simulink model "task4-Simulink"  (R2015b)
settings: Solver=VariableStepAuto  StartTime=0.0  StopTime=10.0  RelTol=1e-3
values from neighbouring files (symbols this model uses):
  J = 60*10^-7    (= 6e-06)    [All Tasks Compiled.m]
  Kemf = 4.555*10^(-3)*60/(2*pi)    (= 0.043497045947)    [All Tasks Compiled.m]
  Km = 43.5*10^-3    (= 0.0435)    [All Tasks Compiled.m]
  R = 1.45    [All Tasks Compiled.m]
settings Model: Creator=daniella.a  LastModifiedBy=daniella.a

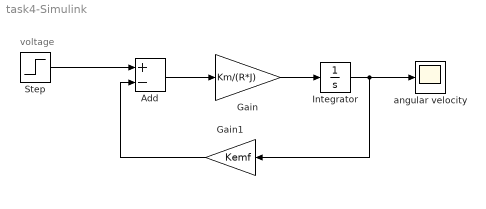
== system task4-Simulink ==
  note: voltage
  Add : Sum  Inputs=+-
  Gain : Gain  Gain=Km/(R*J)
  Gain1 : Gain  Gain=Kemf
  Integrator : Integrator
  Step : Step  Time=0  After=24  SampleTime=0
  angular velocity : Scope
  wires:
  Add/1 -> Gain/1
  Gain/1 -> Integrator/1
  Step/1 -> Add/1
  Integrator/1 -> Gain1/1, angular velocity/1
  Gain1/1 -> Add/2
